simulink model "sched"  (R2022b)
settings: Solver=ode45  StartTime=0.0  StopTime=4.8  RelTol=1e-3  EnableMultiTasking=on
InitFcn:
  | clear functions
libraries: truetime x1
settings Model: Creator=anton  LastModifiedBy=sunan
settings SolverCC: AlgebraicLoopSolver=TrustRegion
settings DataIOCC: SaveFormat=Array  SignalLoggingSaveFormat=ModelDataLogs  ReturnWorkspaceOutputs=off
settings OptimizationCC: BlockReduction=off  BooleanDataType=off  ExpressionDepthLimit=2147483647  LifeSpan=inf
settings DebuggingCC: SaveWithParameterizedLinksMsg=none  UnderspecifiedInitializationDetection=Classic  MergeDetectMultiDrivingBlocksExec=none  SignalResolutionControl=TryResolveAllWithWarning  MultiTaskDSMMsg=warning  MultiTaskCondExecSysMsg=none  FcnCallInpInsideContextMsg=warning  UnconnectedInputMsg=warning  UnconnectedOutputMsg=warning  UnconnectedLineMsg=warning  StateNameClashWarn=warning  SFUnexpectedBacktrackingDiag=warning  SFNoUnconditionalDefaultTransitionDiag=warning  SFExecutionAtInitializationDiag=none  SFMachineParentedDataDiag=warning  ArithmeticOperatorsInVariantConditions=warning
settings HardwareCC: ProdBitPerPointer=32  ProdBitPerSizeT=32  ProdBitPerPtrDiffT=32  ProdLargestAtomicFloat=None  ProdIntDivRoundTo=Undefined  ProdEndianess=Unspecified  ProdWordSize=32  ProdHWDeviceType=32-bit Generic  TargetUnknown=on
settings ModelReferenceCC: EnableRefExpFcnMdlSchedulingChecks=on  PropagateSignalLabelsOutOfModel=off
settings SFSimCC: SimUseLocalCustomCode=off  CustomCodeUndefinedFunction=UseInterfaceOnly
settings RTWCC: RTWUseLocalCustomCode=off  DLArmComputeVersion=19.05
settings CodeAppCC: StateflowObjectComments=on
settings GRTTargetCC: TargetLangStandard=C89/C90 (ANSI)  CombineOutputUpdateFcns=off  GRTInterface=on
settings ConfigComp: CovMetricSettings=dw  CovSaveCumulativeToWorkspaceVar=on  CovSaveSingleToWorkspaceVar=on  CovExternalEMLEnable=off

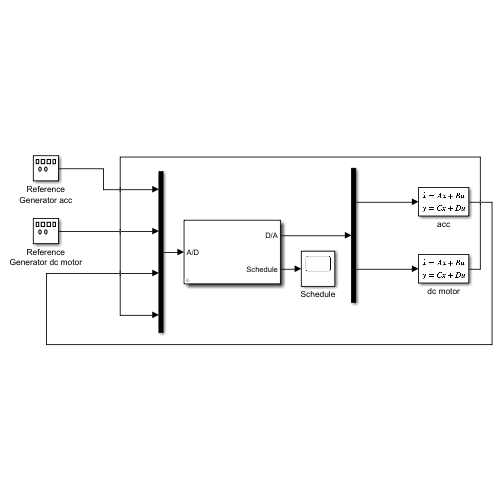
[thumbnail: Simulink's stored preview of the top-level diagram]
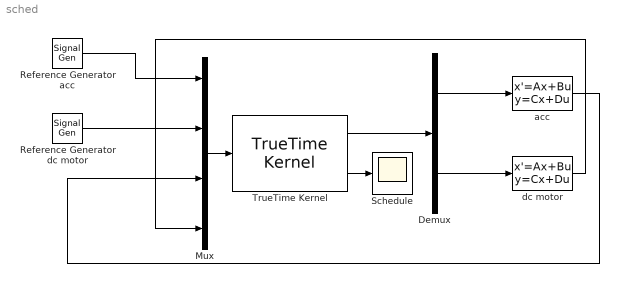
== system sched ==
  Demux : Demux  Outputs=2
      settings: DisplayOption=none
  Mux : Mux
  Reference Generator acc : SignalGenerator  WaveForm=square  Amplitude=-10  Frequency=0.02
  Reference Generator dc motor : SignalGenerator  WaveForm=square  Amplitude=-1  Frequency=0.02
  Schedule : Scope
  TrueTime Kernel : truetime/TrueTime Kernel  sfun=sched_init  args=1  ninputsoutputs=[4 2]  ntriggers=0  trigtype=falling  nwnodenbr=[]  clockoffsetdrift=[0 0]  schedoutput=on  battery=off  poweroutput=off
  acc : StateSpace  A=[0 1; 1 0]  B=[0; 1]  C=[1 0]  D=[0]  InitialCondition=[0;0]
  dc motor : StateSpace  A="[-0.9999    0.9998; -0.0200   -1.9998]"  B=[0.0002;1.9999]  C=[1 0]  D=[0]  InitialCondition=[0;0]
  wires:
  Demux/2 -> dc motor/1
  acc/1 -> Mux/3
  dc motor/1 -> Mux/4
  Mux/1 -> TrueTime Kernel/1
  TrueTime Kernel/1 -> Demux/1
  Demux/1 -> acc/1
  TrueTime Kernel/2 -> Schedule/1
  Reference Generator dc motor/1 -> Mux/2
  Reference Generator acc/1 -> Mux/1
